simulink model "Robot"  (R2025b)
settings: Solver=VariableStepAuto  StartTime=0.0  StopTime=10.0  RelTol=1e-3
libraries: opcualib x1
settings Model: Creator=guilh  LastModifiedBy=guilh

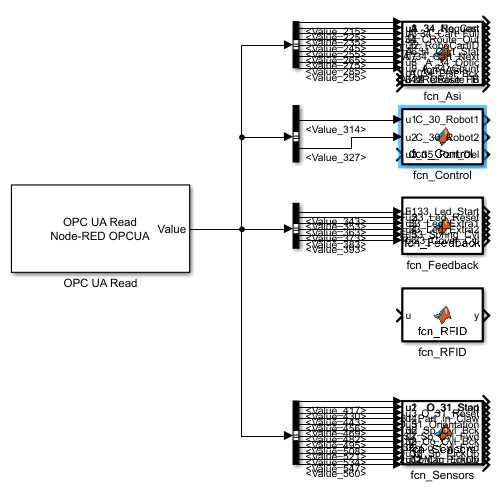
[thumbnail: Simulink's stored preview of the top-level diagram]
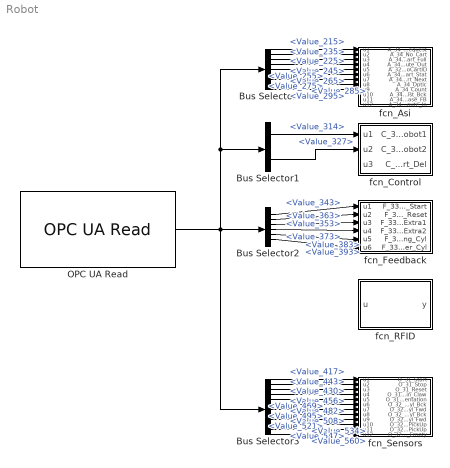
== system Robot ==
  Bus Selector : BusSelector  OutputSignals=Value_215,Value_225,Value_235,Value_245,Value_255,Value_265,Value_275,Value_285,Value_295
  Bus Selector1 : BusSelector  OutputSignals=Value_314,Value_327
  Bus Selector2 : BusSelector  OutputSignals=Value_343,Value_353,Value_363,Value_373,Value_383,Value_393
  Bus Selector3 : BusSelector  OutputSignals=Value_417,Value_430,Value_443,Value_456,Value_469,Value_482,Value_495,Value_508,Value_521,Value_534,Value_547,Value_560
  OPC UA Read : opcualib/OPC UA Read  SelectedServer=Node-RED OPCUA  ServerList=Node-RED OPCUA  NodeList={ '1', 'Value', '6', '215', '1'; '2', 'Value', '6', '225', '1'; '3', 'Value', '6', '235', '1'; '4', 'Value', '6', '245', '1'; '5', 'Value', '6', '255', '1'; '6', 'Value', '6', '265', '1'; '7', 'Value', '6', '275', '1'; '8', 'Value', '6', '285', '1'; '9', 'Value', '6', '295', '1'; '10', 'Value', '6', '314', '1'; '11', 'Value', '6', '327', '1'; '12', 'Value', '6', '343', '1'; '13', 'Value', '6', '353', '1'; '14', 'Value', '6', '363', '1'; '15', 'Value', '6', '373', '1'; '16', 'Value', '6', '383', '1'; '17', 'Value', '6', '393', '1'; '18', 'Value', '6', '417', '1'; '19', 'Value', '6', '430', '1'; '20', 'Value', '6', '443', '1'; '21', 'Value', '6', '456', '1'; '22', 'Value', '6', '469', '1'; '23', 'Value', '6', '482', '1'; '24', 'Value', '6', '495', '1'; '25', 'Value', '6', '508', '1'; '26', 'Value', '6', '521', '1'; '27', 'Value', '6', '534', '1'; '28', 'Value', '6', '547', '1'; '29', 'Value', '6', '560', '1' }  ShowQualityPort=off  ShowTimestampPort=off  ShowTimestampPortAs=Seconds since start  SampleTime=-1
  fcn_Asi : MATLAB Function  TreatAsAtomicUnit=on
  fcn_Control : MATLAB Function  TreatAsAtomicUnit=on
  fcn_Feedback : MATLAB Function  TreatAsAtomicUnit=on
  fcn_RFID : MATLAB Function  TreatAsAtomicUnit=on
  fcn_Sensors : MATLAB Function  TreatAsAtomicUnit=on
  wires:
  OPC UA Read/1 -> Bus Selector3/1, Bus Selector/1, Bus Selector1/1, Bus Selector2/1
  Bus Selector/1 -> fcn_Asi/1(u1)  "<Value_215>"
  Bus Selector/2 -> fcn_Asi/2(u2)  "<Value_225>"
  Bus Selector/3 -> fcn_Asi/3(u3)  "<Value_235>"
  Bus Selector/4 -> fcn_Asi/4(u4)  "<Value_245>"
  Bus Selector/5 -> fcn_Asi/5(u5)  "<Value_255>"
  Bus Selector/6 -> fcn_Asi/6(u6)  "<Value_265>"
  Bus Selector/7 -> fcn_Asi/7(u7)  "<Value_275>"
  Bus Selector/8 -> fcn_Asi/8(u8)  "<Value_285>"
  Bus Selector/9 -> fcn_Asi/9(u9)  "<Value_295>"
  Bus Selector1/1 -> fcn_Control/1(u1)  "<Value_314>"
  Bus Selector1/2 -> fcn_Control/2(u2)  "<Value_327>"
  Bus Selector2/1 -> fcn_Feedback/1(u1)  "<Value_343>"
  Bus Selector2/2 -> fcn_Feedback/2(u2)  "<Value_353>"
  Bus Selector2/3 -> fcn_Feedback/3(u3)  "<Value_363>"
  Bus Selector2/4 -> fcn_Feedback/4(u4)  "<Value_373>"
  Bus Selector2/5 -> fcn_Feedback/5(u5)  "<Value_383>"
  Bus Selector2/6 -> fcn_Feedback/6(u6)  "<Value_393>"
  Bus Selector3/1 -> fcn_Sensors/1(u1)  "<Value_417>"
  Bus Selector3/2 -> fcn_Sensors/2(u2)  "<Value_430>"
  Bus Selector3/3 -> fcn_Sensors/3(u3)  "<Value_443>"
  Bus Selector3/4 -> fcn_Sensors/4(u4)  "<Value_456>"
  Bus Selector3/5 -> fcn_Sensors/5(u5)  "<Value_469>"
  Bus Selector3/6 -> fcn_Sensors/6(u6)  "<Value_482>"
  Bus Selector3/7 -> fcn_Sensors/7(u7)  "<Value_495>"
  Bus Selector3/8 -> fcn_Sensors/8(u8)  "<Value_508>"
  Bus Selector3/9 -> fcn_Sensors/9(u9)  "<Value_521>"
  Bus Selector3/10 -> fcn_Sensors/10(u10)  "<Value_534>"
  Bus Selector3/11 -> fcn_Sensors/11(u11)  "<Value_547>"
  Bus Selector3/12 -> fcn_Sensors/12(u12)  "<Value_560>"

== matlab function Robot/fcn_RFID ==
  data: u input; y output
function y = fcn_RFID(u)

y = u;

== matlab function Robot/fcn_Control ==
  data: u1 input; C_30_Robot1 output; u2 input; C_30_Robot2 output; u3 input; C_35_Part_Del output
function [C_30_Robot1,C_30_Robot2,C_35_Part_Del] = fcn_Control(u1,u2,u3)

C_30_Robot1 = u1;
C_30_Robot2 = u2;
C_35_Part_Del = u3;

== matlab function Robot/fcn_Asi ==
  data: u1 input; A_34_Request output; u2 input; u3 input; u4 input; u5 input; u6 input; u7 input; u8 input; u9 input; A_34_No_Cart output; A_34_Cart_Full output; A_34_CRoute_Out output; A_32_RoboCartID output; A_34_Cart_Stat output; A_34_Cart_Next output; A_34_Optic output; A_34_Count output; A_34_Pist_Bck output; A_34_Release_FB output; u10 input; u11 input; u12 input; A_34_CRoute_In output
function [A_34_Request,A_34_No_Cart,A_34_Cart_Full,A_34_CRoute_Out,...
A_32_RoboCartID,A_34_Cart_Stat,A_34_Cart_Next,A_34_Optic,A_34_Count,...
A_34_Pist_Bck,A_34_Release_FB,A_34_CRoute_In]... 
= fcn_Asi(u1,u2,u3,u4,u5,u6,u7,u8,u9,u10,u11,u12)

A_34_Request = u1;
A_34_No_Cart = u2;
A_34_Cart_Full = u3;
A_34_CRoute_Out = u4;
A_32_RoboCartID = u5;
A_34_Cart_Stat = u6;
A_34_Cart_Next = u7;
A_34_Optic = u8;
A_34_Count = u9;
A_34_Pist_Bck = u10;
A_34_Release_FB = u11;
A_34_CRoute_In = u12;

== matlab function Robot/fcn_Feedback ==
  data: u1 input; F_33_Led_Start output; u2 input; u3 input; u4 input; u5 input; u6 input; F_33_Led_Reset output; F_33_Led_Extra1 output; F_33_Led_Extra2 output; F_33_Spring_Cyl output; F_33_Cover_Cyl output
function [F_33_Led_Start,F_33_Led_Reset,...
    F_33_Led_Extra1,F_33_Led_Extra2,...
    F_33_Spring_Cyl,F_33_Cover_Cyl] = fcn_Feedback(u1,u2,u3,u4,u5,u6)

F_33_Led_Start = u1
F_33_Led_Reset = u2
F_33_Led_Extra1 = u3
F_33_Led_Extra2 = u4
F_33_Spring_Cyl = u5
F_33_Cover_Cyl = u6

== matlab function Robot/fcn_Sensors ==
  data: u1 input; O_31_Start output; u2 input; u3 input; u4 input; u5 input; u6 input; u7 input; u8 input; u9 input; u10 input; u11 input; u12 input; O_31_Stop output; O_31_Reset output; O_31_Part_in_Claw output; O_31_Orientation output; O_32_Sp_Cyl_Bck output; O_32_Sp_Cyl_Fwd output; O_32_Co_Cyl_Bck output; O_32_Co_Cyl_Fwd output; O_32_Sp_PickUp output; O_32_Co_PickUp output; O_32_CoMag_Empty output
function [O_31_Start,...
    O_31_Stop,O_31_Reset,...
    O_31_Part_in_Claw,O_31_Orientation,...
    O_32_Sp_Cyl_Bck,O_32_Sp_Cyl_Fwd,...
    O_32_Co_Cyl_Bck,O_32_Co_Cyl_Fwd,...
    O_32_Sp_PickUp,O_32_Co_PickUp,...
    O_32_CoMag_Empty] = fcn_Sensors(u1,u2,u3,u4,u5,u6,u7,u8,u9,u10,u11,u12)

O_31_Start = u1
O_31_Stop = u2
O_31_Reset = u3
O_31_Part_in_Claw = u4
O_31_Orientation = u5
O_32_Sp_Cyl_Bck = u6
O_32_Sp_Cyl_Fwd = u7
O_32_Co_Cyl_Bck = u8
O_32_Co_Cyl_Fwd = u9
O_32_Sp_PickUp = u10
O_32_Co_PickUp = u11
O_32_CoMag_Empty = u12
